simulink model "PID_only_using_distance"  (R2024b)
settings: Solver=FixedStepAuto  StartTime=0.0  StopTime=60  RelTol=1e-3
libraries: slpidlib x1
settings Model: Creator=Corné  LastModifiedBy=Corné

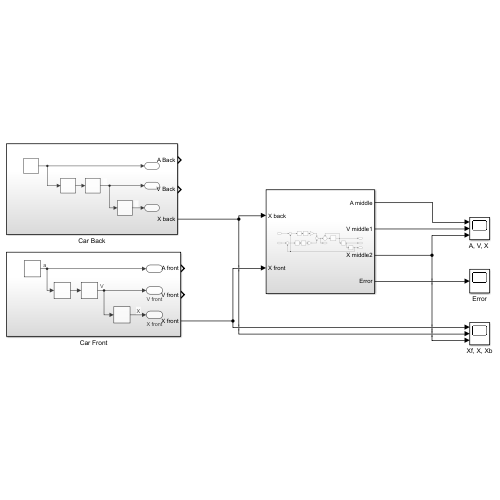
[thumbnail: Simulink's stored preview of the top-level diagram]
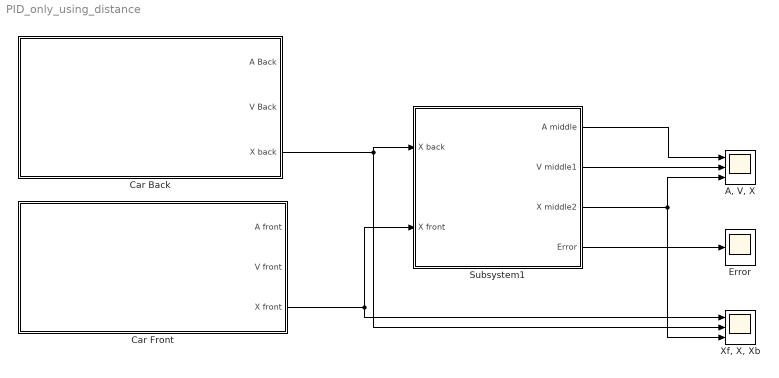
== system PID_only_using_distance ==
  "A, V, X " : Scope  NumInputPorts=3
  Car Back : Subsystem
  Car Front : Subsystem
  Error : Scope
  Subsystem1 : Subsystem
  "Xf, X, Xb" : Scope  NumInputPorts=3
  wires:
  Car Front/3(X front) -> "Xf, X, Xb"/1, Subsystem1/2(X front)
  Car Back/3(X back) -> Subsystem1/1("X back "), "Xf, X, Xb"/2
  Subsystem1/1(A middle) -> "A, V, X "/1
  Subsystem1/2(V middle1) -> "A, V, X "/2
  Subsystem1/3(X middle2) -> "A, V, X "/3, "Xf, X, Xb"/3
  Subsystem1/4(Error) -> Error/1

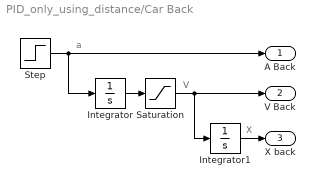
== system PID_only_using_distance/Car Back ==
  note: X
  note: V
  note: a
  Integrator : Integrator  InitialCondition=50
  Integrator1 : Integrator
  Saturation : Saturate  UpperLimit=50  LowerLimit=-50
  Step : Step  Time=0  SampleTime=0
  A Back : Outport
  V Back : Outport  Port=2
  X back : Outport  Port=3
  wires:
  Integrator/1 -> Saturation/1
  Step/1 -> Integrator/1, A Back/1
  Integrator1/1 -> X back/1
  Saturation/1 -> Integrator1/1, V Back/1

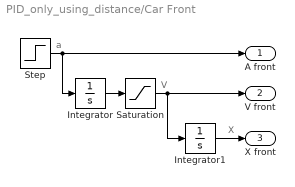
== system PID_only_using_distance/Car Front ==
  note: X
  note: V
  note: a
  Integrator : Integrator  InitialCondition=50
  Integrator1 : Integrator  InitialCondition=40
  Saturation : Saturate  UpperLimit=50  LowerLimit=-50
  Step : Step  Time=0  SampleTime=0
  A front : Outport
  V front : Outport  Port=2
  X front : Outport  Port=3
  wires:
  Integrator/1 -> Saturation/1
  Step/1 -> A front/1, Integrator/1
  Integrator1/1 -> X front/1
  Saturation/1 -> V front/1, Integrator1/1

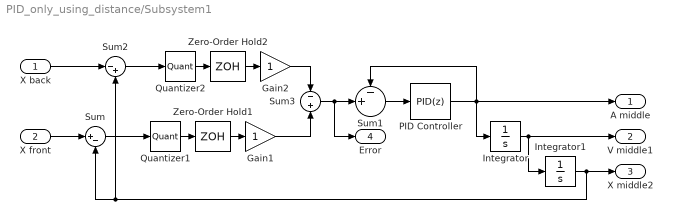
== system PID_only_using_distance/Subsystem1 ==
  "X back " : Inport
  X front : Inport  Port=2
  Gain1 : Gain
  Gain2 : Gain
  Integrator : Integrator  InitialCondition=40
  Integrator1 : Integrator  InitialCondition=30
  PID Controller : slpidlib/PID Controller  Controller=PID  Form=Parallel  TimeDomain=Discrete-time  UseExternalTs=off  SampleTime=-1  IntegratorMethod=Forward Euler  FilterMethod=Forward Euler  ControllerParametersSource=internal  P=0.2  I=0  UseKiTs=off  D=0.6  UseExternalDerivativeSource=off  N=100  UseFilter=on  TunerSelectOption=Transfer Function Based (PID Tuner App)  InitialConditionSource=internal  InitialConditionForIntegrator=0  InitialConditionForFilter=0  DifferentiatorICPrevScaledInput=0  ExternalReset=none  TrackingMode=off  Kt=1  LimitOutput=off  SatLimitsSource=internal  UpperSaturationLimit=inf  LowerSaturationLimit=-inf  LinearizeAsGain=on  AntiWindupMode=none  Kb=1  LimitIntegrator=off  UpperIntegratorSaturationLimit=inf  LowerIntegratorSaturationLimit=-inf  POutMin=[]  POutMax=[]  IOutMin=[]  IOutMax=[]  DOutMin=[]  DOutMax=[]  NOutMin=[]  NOutMax=[]  SumOutMin=[]  SumOutMax=[]  SaturationOutMin=[]  SaturationOutMax=[]  PParamMin=[]  PParamMax=[]  IParamMin=[]  IParamMax=[]  DParamMin=[]  DParamMax=[]  NParamMin=[]  NParamMax=[]  KbParamMin=[]  KbParamMax=[]  KtParamMin=[]  KtParamMax=[]  KbOutMin=[]  KbOutMax=[]  KtOutMin=[]  KtOutMax=[]  IntegratorOutMin=[]  IntegratorOutMax=[]  FilterOutMin=[]  FilterOutMax=[]  SumI1OutMin=[]  SumI1OutMax=[]  SumI2OutMin=[]  SumI2OutMax=[]  SumI3OutMin=[]  SumI3OutMax=[]  SumI4OutMin=[]  SumI4OutMax=[]  SumDOutMin=[]  SumDOutMax=[]  DifferentiatorOutMin=[]  DifferentiatorOutMax=[]  FilterDiffOutCoefMin=[]  FilterDiffOutCoefMax=[]  ReciprocalOutMin=[]  ReciprocalOutMax=[]  SumDenOutMin=[]  SumDenOutMax=[]  SumNumOutMin=[]  SumNumOutMax=[]  DivideOutMin=[]  DivideOutMax=[]  UdiffTsProdOutMin=[]  UdiffTsProdOutMax=[]  NTsProdOutMin=[]  NTsProdOutMax=[]  UintegralTsProdOutMin=[]  UintegralTsProdOutMax=[]  UngainTsProdOutMin=[]  UngainTsProdOutMax=[]  ClampingZeroOutDataTypeStr=Inherit: Inherit via back propagation  ClampingZeroOutMin=[]  ClampingZeroOutMax=[]  FilterDenConstantOutDataTypeStr=Inherit: Inherit via back propagation  FilterDenConstantOutMin=[]  FilterDenConstantOutMax=[]  PCopyOutDataTypeStr=Inherit: Inherit via back propagation  PCopyOutMin=[]  PCopyOutMax=[]  NCopyOutDataTypeStr=Inherit: Inherit via back propagation  NCopyOutMin=[]  NCopyOutMax=[]  IntegratorContinuousStateAttributes=''  IntegratorStateMustResolveToSignalObject=off  IntegratorRTWStateStorageClass=Auto  FilterContinuousStateAttributes=''  FilterStateMustResolveToSignalObject=off  FilterRTWStateStorageClass=Auto  ParallelPVariant=InternalParameters  IdealPVariant=Disabled  IVariant=InternalParameters  DVariant=InternalParameters  IntegratorVariant=Discrete  SatVariant=Disabled  AWVariant=Passthrough  PCopyVariant=Disabled  TRVariant=Disabled  FdbkBlocksVariant=Forward  IdealPFdbkVariant=Disabled  SatFdbkVariant=Disabled  DerivativeFilterVariant=ForwardEulerFilter  NVariant=InternalParameters  NCopyVariant=Disabled  FilterICVariant=InternalICsFilter  IntegratorICVariant=InternalICs  ExternalResetVariant=Disabled  TRSumVariant=Passthrough  SumFdbkVariant=Disabled  SumVariant=Sum_PID  TsampFilterVariant=InternalTs  TsampNgainVariant=Passthrough  TsampIntegralVariant=Disabled_SignalSpec  ExternalSaturationOutDataTypeStr=Inherit: Same as second input  DerivativeSourceVariant=ErrorSignal  PreIntVariant=InternalPreInt
  Quantizer1 : Quantizer  QuantizationInterval=0.1
  Quantizer2 : Quantizer  QuantizationInterval=0.1
  Sum : Sum  Inputs=|+-
  Sum1 : Sum  Inputs=-+|
  Sum2 : Sum  Inputs=|-+
  Sum3 : Sum  Inputs=-|+
  Zero-Order Hold1 : ZeroOrderHold  SampleTime=0.1
  Zero-Order Hold2 : ZeroOrderHold  SampleTime=0.1
  A middle : Outport
  V middle1 : Outport  Port=2
  X middle2 : Outport  Port=3
  Error : Outport  Port=4
  wires:
  Integrator/1 -> Integrator1/1, V middle1/1
  Integrator1/1 -> Sum/2, Sum2/2, X middle2/1
  Sum1/1 -> PID Controller/1
  PID Controller/1 -> Sum1/1, Integrator/1, A middle/1
  X front/1 -> Sum/1
  "X back "/1 -> Sum2/1
  Sum3/1 -> Error/1, Sum1/2
  Quantizer1/1 -> Zero-Order Hold1/1
  Zero-Order Hold1/1 -> Gain1/1
  Sum/1 -> Quantizer1/1
  Gain1/1 -> Sum3/2
  Quantizer2/1 -> Zero-Order Hold2/1
  Zero-Order Hold2/1 -> Gain2/1
  Sum2/1 -> Quantizer2/1
  Gain2/1 -> Sum3/1
